simulink model "amplifierboard"  (R2020b)
settings: Solver=FixedStepDiscrete  StartTime=0.0  StopTime=2  FixedStep=0.01  RelTol=1e-3
InitFcn:
  | mbd_s32k_consistency_checks(bdroot(gcs));
undefined symbols (not defined in the file): AutoLowerVal, AutoRaiseVal, HoldVal, LED_En, LED_Off, LED_On, Logic_High, Logic_Low, LQFP, ManualLowerVal, ManualRaiseVal, PWRWNDW_CHDLCK, sC_bool_PWMEN, sC_cnt_FWSetting, sC_cnt_Mtr_DrvNo_HB, sC_cnt_PWMHB1to4, sC_cnt_PWMHB5to8, sC_cnt_TargetSlowRange, sC_pct_ManualMax, sC_pct_RampDwn, sC_pct_RampUp, sC_pct_StartPWM, sC_pct_Targetmax, SwitchPackRangeOffset, Threshold_Value, Tolerant_Time
libraries: mbd_s32k1xx_ec_toolbox x205, simulink x59, canmsglib x19, Filter x15, wndwcmd x3
(part 3 of 6)

== system amplifierboard/Initialization- Memory Defines/Generate_Data2 ==
  Constant2 : Constant  Value=3  OutDataTypeStr=uint8
  Constant{3,5..6,8} (4 alike) : Constant  Value=2  OutDataTypeStr=uint8
  Constant4 : Constant  OutDataTypeStr=uint8
  Constant7 : Constant  OutDataTypeStr=uint8
  Data Store Read1 : DataStoreRead  DataStoreName=data2
  Mux : Mux  Inputs=8
  Width : Width  DataType=uint8
  Data : Outport
  Length : Outport  Port=2
  wires:
  Mux/1 -> Width/1, Data/1
  Constant2/1 -> Mux/1
  Constant3/1 -> Mux/2
  Constant5/1 -> Mux/4
  Data Store Read1/1 -> Mux/5
  Constant4/1 -> Mux/3
  Constant6/1 -> Mux/6
  Constant7/1 -> Mux/7
  Constant8/1 -> Mux/8
  Width/1 -> Length/1

== system amplifierboard/Initialization- Memory Defines/Generate_Data3 ==
  Constant2 : Constant  Value=3  OutDataTypeStr=uint8
  Constant{3,5..6,8} (4 alike) : Constant  Value=2  OutDataTypeStr=uint8
  Constant4 : Constant  OutDataTypeStr=uint8
  Constant7 : Constant  OutDataTypeStr=uint8
  Data Store Read1 : DataStoreRead  DataStoreName=data3
  Mux : Mux  Inputs=8
  Width : Width  DataType=uint8
  Data : Outport
  Length : Outport  Port=2
  wires:
  Mux/1 -> Width/1, Data/1
  Constant2/1 -> Mux/1
  Constant3/1 -> Mux/2
  Constant5/1 -> Mux/4
  Data Store Read1/1 -> Mux/5
  Constant4/1 -> Mux/3
  Constant6/1 -> Mux/6
  Constant7/1 -> Mux/7
  Constant8/1 -> Mux/8
  Width/1 -> Length/1

== system amplifierboard/Initialization- Memory Defines/Generate_Data4 ==
  Constant2 : Constant  Value=3  OutDataTypeStr=uint8
  Constant{3,5..6,8} (4 alike) : Constant  Value=2  OutDataTypeStr=uint8
  Constant4 : Constant  OutDataTypeStr=uint8
  Constant7 : Constant  OutDataTypeStr=uint8
  Data Store Read1 : DataStoreRead  DataStoreName=data5
  Mux : Mux  Inputs=8
  Width : Width  DataType=uint8
  Data : Outport
  Length : Outport  Port=2
  wires:
  Width/1 -> Length/1
  Constant8/1 -> Mux/8
  Constant7/1 -> Mux/7
  Constant6/1 -> Mux/6
  Constant4/1 -> Mux/3
  Data Store Read1/1 -> Mux/5
  Constant5/1 -> Mux/4
  Constant3/1 -> Mux/2
  Constant2/1 -> Mux/1
  Mux/1 -> Data/1, Width/1

== system amplifierboard/Initialization- Memory Defines/Generate_Data5 ==
  Constant2 : Constant  Value=3  OutDataTypeStr=uint8
  Constant{3,5..6,8} (4 alike) : Constant  Value=2  OutDataTypeStr=uint8
  Constant4 : Constant  OutDataTypeStr=uint8
  Constant7 : Constant  OutDataTypeStr=uint8
  Data Store Read1 : DataStoreRead  DataStoreName=data4
  Mux : Mux  Inputs=8
  Width : Width  DataType=uint8
  Data : Outport
  Length : Outport  Port=2
  wires:
  Mux/1 -> Width/1, Data/1
  Constant2/1 -> Mux/1
  Constant3/1 -> Mux/2
  Constant5/1 -> Mux/4
  Data Store Read1/1 -> Mux/5
  Constant4/1 -> Mux/3
  Constant6/1 -> Mux/6
  Constant7/1 -> Mux/7
  Constant8/1 -> Mux/8
  Width/1 -> Length/1

== system amplifierboard/Initialization- Memory Defines/Generate_Data6 ==
  Constant2 : Constant  Value=3  OutDataTypeStr=uint8
  Constant{3,5..6,8} (4 alike) : Constant  Value=2  OutDataTypeStr=uint8
  Constant4 : Constant  OutDataTypeStr=uint8
  Constant7 : Constant  OutDataTypeStr=uint8
  Data Store Read1 : DataStoreRead  DataStoreName=data6
  Mux : Mux  Inputs=8
  Width : Width  DataType=uint8
  Data : Outport
  Length : Outport  Port=2
  wires:
  Mux/1 -> Width/1, Data/1
  Constant2/1 -> Mux/1
  Constant3/1 -> Mux/2
  Constant5/1 -> Mux/4
  Data Store Read1/1 -> Mux/5
  Constant4/1 -> Mux/3
  Constant6/1 -> Mux/6
  Constant7/1 -> Mux/7
  Constant8/1 -> Mux/8
  Width/1 -> Length/1

== system amplifierboard/Initialization- Memory Defines/Generate_Data7 ==
  Constant2 : Constant  OutDataTypeStr=uint8
  Constant3 : Constant  OutDataTypeStr=uint8
  Constant{4..8} (5 alike) : Constant  Value=85  OutDataTypeStr=uint8
  Data Store Read1 : DataStoreRead  DataStoreName=data6
  Mux : Mux  Inputs=8
  Width : Width  DataType=uint8
  Data : Outport
  Length : Outport  Port=2
  wires:
  Mux/1 -> Width/1, Data/1
  Constant2/1 -> Mux/1
  Constant3/1 -> Mux/2
  Constant5/1 -> Mux/4
  Data Store Read1/1 -> Mux/5
  Constant4/1 -> Mux/3
  Constant6/1 -> Mux/6
  Constant7/1 -> Mux/7
  Constant8/1 -> Mux/8
  Width/1 -> Length/1

== system amplifierboard/Initialization- Memory Defines/Subsystem ==
  FLASH_Config : mbd_s32k1xx_ec_toolbox/Core and System Blocks/FLASH Blocks/FLASH_Config  depart=0x2  eeesize=4096  csec_en=off  csec_num_user_keys=5 keys
  FLASH_EEERead : mbd_s32k1xx_ec_toolbox/Core and System Blocks/FLASH Blocks/FLASH_EEERead  base=0x14000000  offset=0x0F00  ptr=uint16_t
  FLASH_EEERead6 : mbd_s32k1xx_ec_toolbox/Core and System Blocks/FLASH Blocks/FLASH_EEERead  base=0x14000000  offset=0x0F0C  ptr=uint16_t
  If : If  NumInputs=2  IfExpression=(u1 <= 1200) & (u2 <= 750)
  If Action Subsystem : Subsystem  TreatAsAtomicUnit=on
  If Action Subsystem1 : Subsystem  TreatAsAtomicUnit=on  mask{sC_WindSw_NormOpen=1072, sC_WindSw_Dwn=680, sC_WindSw_ExpDwn=437, sC_WindSw_Up=257, sC_WindSw_ExpUp=114}
  wires:
  If/2 -> If Action Subsystem1/Action
  If/1 -> If Action Subsystem/Action
  FLASH_EEERead/1 -> If/1
  FLASH_EEERead6/1 -> If/2

== system amplifierboard/Motor_Control/Motor_Control ==
  note: MotorDir Index
      | Motor
      | Driver
      | HB
      | DRV_SO
      |
      | PWM
      | PWM_Pin
      | PWM FTM CH
      |
      | 1
      | Motor1
      | DRV1
      | 1,2
      | DRV1_SO_1
      |
      | DRV1_PWM1
      | PTA17
      | FTM0_CH6
      |
      | 2
      | Motor2
      | DRV1
      | 3,4
      | DRV1_SO_2
      |
      | DRV1_PWM2
      | PTA11
      | FTM1_CH5
      |
      | 3
      | Motor3
      | DRV1
      | 5,6
      | DRV2_SO_2
      |
      | DRV1_PWM3
      | PTA12
      | FTM1_CH6
      |
      | 4
      | Motor4
      | DRV1
      | 7,8
      | DRV2_SO_1
      |
      | DRV1_PWM4
      | PTA13
      | FTM1_CH7
      |
      | 5
      | Motor5
      | DRV2
      | 1,2
      | DRV3_SO_2
      |
      | DRV2_PWM1
      | PTB17
      | FTM0_CH5
      |
      | 6
      | Motor6
      | DRV2
      | 3,4
      | DRV3_SO_1
      |
      | DRV2_PWM2
      | PTB9
      | FTM3_CH1
      |
      | Shared Channels -None
  cMM_aV_int_MotorDir : Inport  OutDataTypeStr=int8  PortDimensions=6
  BRAKE1 : mbd_s32k1xx_ec_toolbox/GPIO Blocks/Digital_Output  gpio_pin=PTA8: [PTA8 | Port A I/O]  init_val=High  drive_strength=High
  BRAKE2 : mbd_s32k1xx_ec_toolbox/GPIO Blocks/Digital_Output  gpio_pin=PTA0: [PTA0 | Port A I/O]  init_val=High  drive_strength=High
  Chart : Stateflow chart  TreatAsAtomicUnit=on
  Constant : Constant  Value=sC_cnt_PWMHB1to4
  Constant1 : Constant  Value=sC_cnt_PWMHB5to8
  Constant2 : Constant  Value=sC_cnt_Mtr_DrvNo_HB
  Constant3 : Constant  Value=sC_bool_PWMEN
  Constant4 : Constant  Value=sC_cnt_FWSetting  OutDataTypeStr=uint8
  Constant{5..8} (4 alike) : Constant  OutDataTypeStr=Inherit: Inherit via back propagation
  Digital_Output : mbd_s32k1xx_ec_toolbox/GPIO Blocks/Digital_Output  gpio_pin=PTE0: [PTE0 | Port E I/O]  init_val=High  drive_strength=High
  Digital_Output1 : mbd_s32k1xx_ec_toolbox/GPIO Blocks/Digital_Output  gpio_pin=PTB8: [PTB8 | Port B I/O]  init_val=High  drive_strength=High
  "LPSPI_Config " : mbd_s32k1xx_ec_toolbox/Communication Blocks/SPI Blocks/LPSPI_Config   Priority=0  InstanceNumber=2  Role=Master  BaudRate=10000  ShowAdvanced=on  sin=PTC0: [LPSPI2_SIN | LPSPI Serial Data Input]  sout=PTC1: [LPSPI2_SOUT | LPSPI Serial Data Output]  sck=PTC15: [LPSPI2_SCK | LPSPI Serial Clock I/O]  pcs0=PTE11: [LPSPI2_PCS0 | Peripheral Chip Select 0]  pcs1=None  pcs2=None  pcs3=None  CPHA=1  CPOL=0  BitOrder=MSB first  TransferSize=8  WhichPCS=0  PCSPol=ActiveLow  ContinuousTransfer=on
  LPSPI_Config 1 : mbd_s32k1xx_ec_toolbox/Communication Blocks/SPI Blocks/LPSPI_Config   Priority=0  InstanceNumber=1  Role=Master  BaudRate=10000  ShowAdvanced=on  sin=PTD1: [LPSPI1_SIN | LPSPI Serial Data Input]  sout=PTB16: [LPSPI1_SOUT | LPSPI Serial Data Output]  sck=PTD0: [LPSPI1_SCK | LPSPI Serial Clock I/O]  pcs0=None  pcs1=PTA6: [LPSPI1_PCS1 | Peripheral Chip Select 1]  pcs2=None  pcs3=None  CPHA=1  CPOL=0  BitOrder=MSB first  TransferSize=8  WhichPCS=0  PCSPol=ActiveLow  ContinuousTransfer=on
  nSLEEP1 : mbd_s32k1xx_ec_toolbox/GPIO Blocks/Digital_Output  gpio_pin=PTA9: [PTA9 | Port A I/O]  init_val=High  drive_strength=High
  nSLEEP2 : mbd_s32k1xx_ec_toolbox/GPIO Blocks/Digital_Output  gpio_pin=PTA1: [PTA1 | Port A I/O]  init_val=High  drive_strength=High
  8718_FailSafe : Outport
  MotorDriverState : Outport  Port=2
  wires:
  Chart/1(DRV1_OFF) -> Digital_Output/1
  Chart/2(DRV2_OFF) -> Digital_Output1/1
  Constant/1 -> Chart/2(sC_cnt_PWMHB1to4)
  Constant1/1 -> Chart/3(sC_cnt_PWMHB5to8)
  Constant2/1 -> Chart/4(sC_cnt_Mtr_DrvNo_HB)
  Constant3/1 -> Chart/5(sC_bool_PWMEN)
  Constant4/1 -> Chart/6(sC_cnt_FWSetting)
  cMM_aV_int_MotorDir/1 -> Chart/1(aV_int_MotorDir)
  Constant7/1 -> nSLEEP1/1
  Constant6/1 -> BRAKE2/1
  Constant8/1 -> nSLEEP2/1
  Constant5/1 -> BRAKE1/1
  Chart/3(FailSafe) -> 8718_FailSafe/1
  Chart/4(MotorDriverState) -> MotorDriverState/1

== system amplifierboard/Motor_Control/Subsystem ==
  note: MotorDir Index
      | Motor
      | Driver
      | HB
      | DRV_SO
      |
      | PWM
      | PWM_Pin
      | PWM FTM CH
      |
      | 1
      | Motor1
      | DRV1
      | 1,2
      | DRV1_SO_1
      |
      | DRV1_PWM1
      | PTA17
      | FTM0_CH6
      |
      | 2
      | Motor2
      | DRV1
      | 3,4
      | DRV1_SO_2
      |
      | DRV1_PWM2
      | PTA11
      | FTM1_CH5
      |
      | 3
      | Motor3
      | DRV1
      | 5,6
      | DRV2_SO_2
      |
      | DRV1_PWM3
      | PTA12
      | FTM1_CH6
      |
      | 4
      | Motor4
      | DRV1
      | 7,8
      | DRV2_SO_1
      |
      | DRV1_PWM4
      | PTA13
      | FTM1_CH7
      |
      | 5
      | Motor5
      | DRV2
      | 1,2
      | DRV3_SO_2
      |
      | DRV2_PWM1
      | PTB17
      | FTM0_CH5
      |
      | 6
      | Motor6
      | DRV2
      | 3,4
      | DRV3_SO_1
      |
      | DRV2_PWM2
      | PTB9
      | FTM3_CH1
      |
      | Shared Channels -None
  cMM_aV_int_MotorDir1 : Inport  OutDataTypeStr=int8  PortDimensions=6
  cMM_aV_int_PositionError : Inport  Port=2  OutDataTypeStr=uint8  PortDimensions=6
  Abs : Abs
  Chart : Stateflow chart  TreatAsAtomicUnit=on
  Constant : Constant  Value=sC_pct_RampUp  OutDataTypeStr=single
  Constant1 : Constant  Value=sC_pct_RampDwn  OutDataTypeStr=single
  Constant2 : Constant  Value=sC_pct_StartPWM  OutDataTypeStr=single
  Constant3 : Constant  Value=sC_pct_ManualMax  OutDataTypeStr=single
  Constant4 : Constant  Value=sC_pct_Targetmax  OutDataTypeStr=single
  Constant5 : Constant  Value=sC_cnt_TargetSlowRange  OutDataTypeStr=uint16
  aV_pct_PWMOut1 : Outport  OutDataTypeStr=single  PortDimensions=6
  wires:
  Abs/1 -> Chart/1(aV_int_MotorDir)
  Constant1/1 -> Chart/4(RampDwn)
  Constant3/1 -> Chart/6(ManualMaxPWM)
  Constant4/1 -> Chart/7(TargetMaxPWM)
  Constant5/1 -> Chart/8(TargetSlowRange)
  Constant2/1 -> Chart/5(StartPWM)
  cMM_aV_int_MotorDir1/1 -> Abs/1
  Constant/1 -> Chart/3(RampUp)
  Chart/1(PWM_Out) -> aV_pct_PWMOut1/1
  cMM_aV_int_PositionError/1 -> Chart/2(PositionError)

== system amplifierboard/TC1047A_Module/temperature_conversion ==
  In1 : Inport
  Constant1 : Constant  Value=273
  Data Type Conversion : DataTypeConversion
  Degree_to_Kelvin : Sum
  Divide : Product  Inputs=*/  RndMeth=Zero  SaturateOnIntegerOverflow=on
  Divide1 : Product  Inputs=*/  RndMeth=Zero  SaturateOnIntegerOverflow=on
  Divide2 : Product  Inputs=**  RndMeth=Zero  SaturateOnIntegerOverflow=on
  Subtract : Sum  Inputs=+-
  adc_resolution_val : Constant  Value=4095
  adc_vref_val : Constant  Value=5
  mv_to_temp_factor_val : Constant  Value=0.01
  temp_offset_factor_val : Constant  Value=0.5
  AmpBoard_PRV_CAN_Msg_TX_TMP : Outport
  wires:
  Subtract/1 -> Divide/1
  Divide2/1 -> Subtract/1
  In1/1 -> Data Type Conversion/1
  adc_resolution_val/1 -> Divide1/2
  Data Type Conversion/1 -> Divide1/1
  mv_to_temp_factor_val/1 -> Divide/2
  Divide1/1 -> Divide2/1
  adc_vref_val/1 -> Divide2/2
  temp_offset_factor_val/1 -> Subtract/2
  Divide/1 -> Degree_to_Kelvin/1
  Constant1/1 -> Degree_to_Kelvin/2
  Degree_to_Kelvin/1 -> AmpBoard_PRV_CAN_Msg_TX_TMP/1

== system amplifierboard/CAN_Pack_And_Send/PsngrWndwCntDetect/SwtchPosDetect ==
  SwitchCount : Inport
  FR_Dwn_CntDetect : Subsystem
  FR_ExpDwn_CntDetect : Subsystem
  FR_ExpUp_CntDetect : Subsystem
  FR_NrmOpen_CntDetect : Subsystem
  FR_Up_CntDetect : Subsystem
  SwitchPosDetect : Subsystem
  AvgCount : Outport
  wires:
  FR_NrmOpen_CntDetect/1(HoldCnt) -> SwitchPosDetect/5(HoldCnt)  "HoldCnt"
  SwitchPosDetect/1(AvgCount) -> AvgCount/1  "AvgCount"
  FR_ExpDwn_CntDetect/1(Out) -> SwitchPosDetect/4(AutoLowerCnt)  "AutoLowerCnt"
  FR_Dwn_CntDetect/1(Out1) -> SwitchPosDetect/2(ManLowerCnt)  "ManLowerCnt"
  FR_Up_CntDetect/1(Out3) -> SwitchPosDetect/1(ManRaiseCnt)  "ManRaiseCnt"
  SwitchCount/1 -> FR_Up_CntDetect/1(In3), FR_Dwn_CntDetect/1(In1), FR_ExpUp_CntDetect/1(In2), FR_ExpDwn_CntDetect/1(In), FR_NrmOpen_CntDetect/1(In4), SwitchPosDetect/6(SwitchCount)  "SwitchCount"
  FR_ExpUp_CntDetect/1(AutoRaiseCnt) -> SwitchPosDetect/3(AutoRaiseCnt)

== system amplifierboard/CAN_Pack_And_Send/RLWndwCntDetect/SwtchPosDetect ==
  SwitchCount : Inport
  RL_Dwn_CntDetect : Subsystem
  RL_ExpDwn_CntDetect : Subsystem
  RL_ExpUp_CntDetect : Subsystem
  RL_NrmOpen_CntDetect : Subsystem
  RL_Up_CntDetect : Subsystem
  SwitchPosDetect2 : Subsystem
  AvgCount : Outport
  wires:
  SwitchPosDetect2/1(AvgCount) -> AvgCount/1  "AvgCount"
  SwitchCount/1 -> RL_Up_CntDetect/1(In13), RL_Dwn_CntDetect/1(In11), RL_ExpUp_CntDetect/1(In12), RL_ExpDwn_CntDetect/1(In10), RL_NrmOpen_CntDetect/1(In14), SwitchPosDetect2/6(SwitchCount)
  RL_Up_CntDetect/1(Out13) -> SwitchPosDetect2/1(ManRaiseCnt)  "ManRaiseCnt"
  RL_ExpUp_CntDetect/1(Out12) -> SwitchPosDetect2/3(AutoRaiseCnt)
  RL_Dwn_CntDetect/1(ManLowerCnt) -> SwitchPosDetect2/2(ManLowerCnt)
  RL_ExpDwn_CntDetect/1(AutoLowerCnt) -> SwitchPosDetect2/4(AutoLowerCnt)
  RL_NrmOpen_CntDetect/1(HoldCnt) -> SwitchPosDetect2/5(HoldCnt)

== system amplifierboard/CAN_Pack_And_Send/RRWndwCntDetect/SwtchPosDetect ==
  SwitchCount : Inport
  RR_Dwn_CntDetect : Subsystem
  RR_ExpDwn_CntDetect : Subsystem
  RR_ExpUp_CntDetect : Subsystem
  RR_NrmOpen_CntDetect : Subsystem
  RR_Up_CntDetect : Subsystem
  SwitchPosDetect1 : Subsystem
  AvgCount : Outport
  wires:
  RR_Up_CntDetect/1(Out8) -> SwitchPosDetect1/1(ManRaiseCnt)  "ManRaiseCnt"
  RR_Dwn_CntDetect/1(Out6) -> SwitchPosDetect1/2(ManLowerCnt)  "ManLowerCnt"
  RR_ExpDwn_CntDetect/1(Out5) -> SwitchPosDetect1/4(AutoLowerCnt)  "AutoLowerCnt"
  RR_ExpUp_CntDetect/1(AutoRaiseCnt) -> SwitchPosDetect1/3(AutoRaiseCnt)
  SwitchCount/1 -> RR_Up_CntDetect/1(In8), RR_Dwn_CntDetect/1(In6), RR_ExpUp_CntDetect/1(In7), RR_ExpDwn_CntDetect/1(SwitchCount1), RR_NrmOpen_CntDetect/1(In9), SwitchPosDetect1/6(SwitchCount)
  SwitchPosDetect1/1(AvgCount) -> AvgCount/1  "AvgCount"
  RR_NrmOpen_CntDetect/1(HoldCnt) -> SwitchPosDetect1/5(HoldCnt)

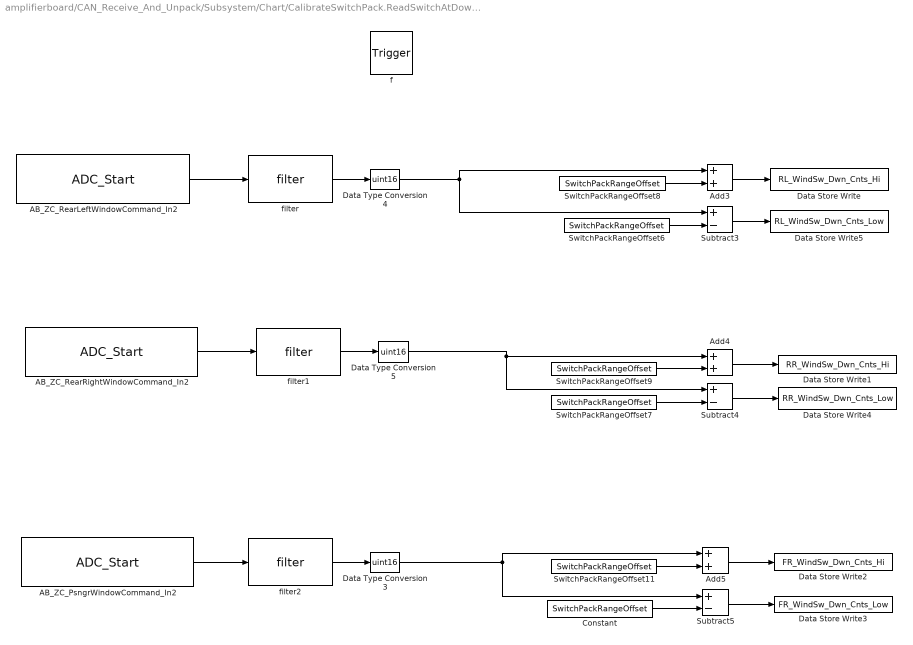
== system amplifierboard/CAN_Receive_And_Unpack/Subsystem/Chart/CalibrateSwitchPack.ReadSwitchAtDownPostion ==
  f : TriggerPort  TriggerType=function-call  VariantControl=(inherit)
      settings: CopyFcn=Stateflow.SLINSF.SimulinkMan.removeBlockPreDeleteFcn  PreDeleteFcn=Stateflow.SLINSF.SimulinkMan.unsafePredeleteFcn
  AB_ZC_PsngrWindowCommand_In2 : mbd_s32k1xx_ec_toolbox/Motor Control Blocks/ADC Blocks/ADC_Start  instance=0  adc_r=A  adc_chan=PTB2: [ADC0_SE6 | ADC Single Ended Input]  aien=off  mcuTargetUpdate=on
  AB_ZC_RearLeftWindowCommand_In2 : mbd_s32k1xx_ec_toolbox/Motor Control Blocks/ADC Blocks/ADC_Start  instance=0  adc_r=A  adc_chan=PTB0: [ADC0_SE4 | ADC Single Ended Input]  aien=off  mcuTargetUpdate=on
  AB_ZC_RearRightWindowCommand_In2 : mbd_s32k1xx_ec_toolbox/Motor Control Blocks/ADC Blocks/ADC_Start  instance=0  adc_r=A  adc_chan=PTB1: [ADC0_SE5 | ADC Single Ended Input]  aien=off  mcuTargetUpdate=on
  Add3 : Sum  OutDataTypeStr=uint16
  Add4 : Sum
  Add5 : Sum
  Constant : Constant  Value=SwitchPackRangeOffset  OutDataTypeStr=uint16
  Data Store Write : DataStoreWrite  DataStoreName=RL_WindSw_Dwn_Cnts_Hi
  Data Store Write1 : DataStoreWrite  DataStoreName=RR_WindSw_Dwn_Cnts_Hi
  Data Store Write2 : DataStoreWrite  DataStoreName=FR_WindSw_Dwn_Cnts_Hi
  Data Store Write3 : DataStoreWrite  DataStoreName=FR_WindSw_Dwn_Cnts_Low
  Data Store Write4 : DataStoreWrite  DataStoreName=RR_WindSw_Dwn_Cnts_Low
  Data Store Write5 : DataStoreWrite  DataStoreName=RL_WindSw_Dwn_Cnts_Low
  Data Type Conversion3 : DataTypeConversion  OutDataTypeStr=uint16
  Data Type Conversion4 : DataTypeConversion  OutDataTypeStr=uint16
  Data Type Conversion5 : DataTypeConversion  OutDataTypeStr=uint16
  Subtract3 : Sum  Inputs=+-
  Subtract4 : Sum  Inputs=+-
  Subtract5 : Sum  Inputs=+-
  SwitchPackRangeOffset{6..9,11} (5 alike) : Constant  Value=SwitchPackRangeOffset  OutDataTypeStr=uint16
  filter : Filter/filter  pwrwndwp_coefcnt=pwrwndwp_coefcnt
  filter1 : Filter/filter  pwrwndwp_coefcnt=pwrwndwp_coefcnt
  filter2 : Filter/filter  pwrwndwp_coefcnt=pwrwndwp_coefcnt
  wires:
  AB_ZC_PsngrWindowCommand_In2/1 -> filter2/1
  AB_ZC_RearRightWindowCommand_In2/1 -> filter1/1
  AB_ZC_RearLeftWindowCommand_In2/1 -> filter/1
  Constant/1 -> Subtract5/2
  SwitchPackRangeOffset11/1 -> Add5/2
  SwitchPackRangeOffset8/1 -> Add3/2
  SwitchPackRangeOffset6/1 -> Subtract3/2
  SwitchPackRangeOffset7/1 -> Subtract4/2
  Add4/1 -> Data Store Write1/1
  SwitchPackRangeOffset9/1 -> Add4/2
  Add5/1 -> Data Store Write2/1
  Subtract3/1 -> Data Store Write5/1
  Add3/1 -> Data Store Write/1
  Subtract4/1 -> Data Store Write4/1
  Subtract5/1 -> Data Store Write3/1
  Data Type Conversion3/1 -> Subtract5/1, Add5/1
  Data Type Conversion4/1 -> Add3/1, Subtract3/1
  Data Type Conversion5/1 -> Subtract4/1, Add4/1
  filter/1 -> Data Type Conversion4/1
  filter1/1 -> Data Type Conversion5/1
  filter2/1 -> Data Type Conversion3/1

== system amplifierboard/CAN_Receive_And_Unpack/Subsystem/Chart/CalibrateSwitchPack.ReadSwitchAtExpDownPosition ==
  f : TriggerPort  TriggerType=function-call  VariantControl=(inherit)
      settings: CopyFcn=Stateflow.SLINSF.SimulinkMan.removeBlockPreDeleteFcn  PreDeleteFcn=Stateflow.SLINSF.SimulinkMan.unsafePredeleteFcn
  AB_ZC_PsngrWindowCommand_In1 : mbd_s32k1xx_ec_toolbox/Motor Control Blocks/ADC Blocks/ADC_Start  instance=0  adc_r=A  adc_chan=PTB2: [ADC0_SE6 | ADC Single Ended Input]  aien=off  mcuTargetUpdate=on
  AB_ZC_RearLeftWindowCommand_In1 : mbd_s32k1xx_ec_toolbox/Motor Control Blocks/ADC Blocks/ADC_Start  instance=0  adc_r=A  adc_chan=PTB0: [ADC0_SE4 | ADC Single Ended Input]  aien=off  mcuTargetUpdate=on
  AB_ZC_RearRightWindowCommand_In1 : mbd_s32k1xx_ec_toolbox/Motor Control Blocks/ADC Blocks/ADC_Start  instance=0  adc_r=A  adc_chan=PTB1: [ADC0_SE5 | ADC Single Ended Input]  aien=off  mcuTargetUpdate=on
  Add1 : Sum
  Add2 : Sum  OutDataTypeStr=uint16
  Add6 : Sum  OutDataTypeStr=uint16
  Data Store Write10 : DataStoreWrite  DataStoreName=RR_WindSw_ExpDwn_Cnts_Hi
  Data Store Write11 : DataStoreWrite  DataStoreName=FR_WindSw_ExpDwn_Cnts_Hi
  Data Store Write6 : DataStoreWrite  DataStoreName=FR_WindSw_ExpDwn_Cnts_Low
  Data Store Write7 : DataStoreWrite  DataStoreName=RR_WindSw_ExpDwn_Cnts_Low
  Data Store Write8 : DataStoreWrite  DataStoreName=RL_WindSw_ExpDwn_Cnts_Hi
  Data Store Write9 : DataStoreWrite  DataStoreName=RL_WindSw_ExpDwn_Cnts_Low
  Data Type Conversion2 : DataTypeConversion  OutDataTypeStr=uint16
  Data Type Conversion3 : DataTypeConversion  OutDataTypeStr=uint16
  Data Type Conversion5 : DataTypeConversion  OutDataTypeStr=uint16
  Subtract1 : Sum  Inputs=+-
  Subtract2 : Sum  Inputs=+-  OutDataTypeStr=uint16
  Subtract6 : Sum  Inputs=+-  OutDataTypeStr=uint16
  SwitchPackRangeOffset1 : Constant  Value=SwitchPackRangeOffset  OutDataTypeStr=uint16
  SwitchPackRangeOffset{3..5,12} (4 alike) : Constant  Value=SwitchPackRangeOffset  OutDataTypeStr=Inherit: Inherit via back propagation
  SwitchPackRangeOffset2 : Constant  Value=SwitchPackRangeOffset  OutDataTypeStr=uint16
  filter : Filter/filter  pwrwndwp_coefcnt=pwrwndwp_coefcnt
  filter1 : Filter/filter  pwrwndwp_coefcnt=pwrwndwp_coefcnt
  filter2 : Filter/filter  pwrwndwp_coefcnt=pwrwndwp_coefcnt
  wires:
  AB_ZC_RearLeftWindowCommand_In1/1 -> filter/1
  AB_ZC_RearRightWindowCommand_In1/1 -> filter1/1
  Subtract6/1 -> Data Store Write6/1
  SwitchPackRangeOffset4/1 -> Subtract2/2
  Subtract1/1 -> Data Store Write9/1
  SwitchPackRangeOffset3/1 -> Subtract1/2
  SwitchPackRangeOffset1/1 -> Subtract6/2
  SwitchPackRangeOffset2/1 -> Add6/2
  Add2/1 -> Data Store Write10/1
  Add6/1 -> Data Store Write11/1
  SwitchPackRangeOffset5/1 -> Add1/2
  Subtract2/1 -> Data Store Write7/1
  SwitchPackRangeOffset12/1 -> Add2/2
  Add1/1 -> Data Store Write8/1
  Data Type Conversion3/1 -> Subtract1/1, Add1/1
  Data Type Conversion2/1 -> Subtract2/1, Add2/1
  Data Type Conversion5/1 -> Add6/1, Subtract6/1
  filter/1 -> Data Type Conversion3/1
  filter1/1 -> Data Type Conversion2/1
  filter2/1 -> Data Type Conversion5/1
  AB_ZC_PsngrWindowCommand_In1/1 -> filter2/1

== system amplifierboard/CAN_Receive_And_Unpack/Subsystem/Chart/CalibrateSwitchPack.ReadSwitchAtExpUpPosition ==
  f : TriggerPort  TriggerType=function-call  VariantControl=(inherit)
      settings: CopyFcn=Stateflow.SLINSF.SimulinkMan.removeBlockPreDeleteFcn  PreDeleteFcn=Stateflow.SLINSF.SimulinkMan.unsafePredeleteFcn
  AB_ZC_PsngrWindowCommand_In4 : mbd_s32k1xx_ec_toolbox/Motor Control Blocks/ADC Blocks/ADC_Start  instance=0  adc_r=A  adc_chan=PTB2: [ADC0_SE6 | ADC Single Ended Input]  aien=off  mcuTargetUpdate=on
  AB_ZC_RearLeftWindowCommand_In4 : mbd_s32k1xx_ec_toolbox/Motor Control Blocks/ADC Blocks/ADC_Start  instance=0  adc_r=A  adc_chan=PTB0: [ADC0_SE4 | ADC Single Ended Input]  aien=off  mcuTargetUpdate=on
  AB_ZC_RearRightWindowCommand_In4 : mbd_s32k1xx_ec_toolbox/Motor Control Blocks/ADC Blocks/ADC_Start  instance=0  adc_r=A  adc_chan=PTB1: [ADC0_SE5 | ADC Single Ended Input]  aien=off  mcuTargetUpdate=on
  Add1 : Sum
  Add2 : Sum
  Add6 : Sum
  Data Store Write12 : DataStoreWrite  DataStoreName=RL_WindSw_ExpUp_Cnts_Low
  Data Store Write2 : DataStoreWrite  DataStoreName=RR_WindSw_ExpUp_Cnts_Hi
  Data Store Write3 : DataStoreWrite  DataStoreName=FR_WindSw_ExpUp_Cnts_Hi
  Data Store Write6 : DataStoreWrite  DataStoreName=FR_WindSw_ExpUp_Cnts_Low
  Data Store Write7 : DataStoreWrite  DataStoreName=RR_WindSw_ExpUp_Cnts_Low
  Data Store Write8 : DataStoreWrite  DataStoreName=RL_WindSw_ExpUp_Cnts_Hi
  Data Type Conversion3 : DataTypeConversion  OutDataTypeStr=uint16
  Data Type Conversion4 : DataTypeConversion  OutDataTypeStr=uint16
  Data Type Conversion6 : DataTypeConversion  OutDataTypeStr=uint16
  Subtract1 : Sum  Inputs=+-
  Subtract2 : Sum  Inputs=+-
  Subtract6 : Sum  Inputs=+-
  SwitchPackRangeOffset{1..5,12} (6 alike) : Constant  Value=SwitchPackRangeOffset  OutDataTypeStr=uint16
  filter : Filter/filter  pwrwndwp_coefcnt=pwrwndwp_coefcnt
  filter1 : Filter/filter  pwrwndwp_coefcnt=pwrwndwp_coefcnt
  filter2 : Filter/filter  pwrwndwp_coefcnt=pwrwndwp_coefcnt
  wires:
  AB_ZC_PsngrWindowCommand_In4/1 -> filter2/1
  AB_ZC_RearRightWindowCommand_In4/1 -> filter1/1
  AB_ZC_RearLeftWindowCommand_In4/1 -> filter/1
  Data Type Conversion6/1 -> Add6/1, Subtract6/1
  Subtract2/1 -> Data Store Write7/1
  SwitchPackRangeOffset5/1 -> Add1/2
  SwitchPackRangeOffset3/1 -> Subtract1/2
  SwitchPackRangeOffset4/1 -> Subtract2/2
  Add1/1 -> Data Store Write8/1
  Data Type Conversion4/1 -> Add2/1, Subtract2/1
  Data Type Conversion3/1 -> Add1/1, Subtract1/1
  SwitchPackRangeOffset2/1 -> Add6/2
  Subtract6/1 -> Data Store Write6/1
  SwitchPackRangeOffset12/1 -> Add2/2
  SwitchPackRangeOffset1/1 -> Subtract6/2
  Add6/1 -> Data Store Write3/1
  Add2/1 -> Data Store Write2/1
  Subtract1/1 -> Data Store Write12/1
  filter/1 -> Data Type Conversion3/1
  filter1/1 -> Data Type Conversion4/1
  filter2/1 -> Data Type Conversion6/1

== system amplifierboard/CAN_Receive_And_Unpack/Subsystem/Chart/CalibrateSwitchPack.ReadSwitchAtNormOpen ==
  f : TriggerPort  TriggerType=function-call  VariantControl=(inherit)
      settings: CopyFcn=Stateflow.SLINSF.SimulinkMan.removeBlockPreDeleteFcn  PreDeleteFcn=Stateflow.SLINSF.SimulinkMan.unsafePredeleteFcn
  AB_ZC_PsngrWindowCommand_In4 : mbd_s32k1xx_ec_toolbox/Motor Control Blocks/ADC Blocks/ADC_Start  instance=0  adc_r=A  adc_chan=PTB2: [ADC0_SE6 | ADC Single Ended Input]  aien=off  mcuTargetUpdate=on
  AB_ZC_RearLeftWindowCommand_In4 : mbd_s32k1xx_ec_toolbox/Motor Control Blocks/ADC Blocks/ADC_Start  instance=0  adc_r=A  adc_chan=PTB0: [ADC0_SE4 | ADC Single Ended Input]  aien=off  mcuTargetUpdate=on
  AB_ZC_RearRightWindowCommand_In4 : mbd_s32k1xx_ec_toolbox/Motor Control Blocks/ADC Blocks/ADC_Start  instance=0  adc_r=A  adc_chan=PTB1: [ADC0_SE5 | ADC Single Ended Input]  aien=off  mcuTargetUpdate=on
  Add : Sum
  Add1 : Sum
  Add2 : Sum
  Data Store Write12 : DataStoreWrite  DataStoreName=RL_WindSw_NrmOpen_Cnts_Low
  Data Store Write13 : DataStoreWrite  DataStoreName=RR_WindSw_NrmOpen_Cnts_Low
  Data Store Write14 : DataStoreWrite  DataStoreName=FR_WindSw_NrmOpen_Cnts_Low
  Data Store Write6 : DataStoreWrite  DataStoreName=FR_WindSw_NrmOpen_Cnts_Hi
  Data Store Write7 : DataStoreWrite  DataStoreName=RR_WindSw_NrmOpen_Cnts_Hi
  Data Store Write8 : DataStoreWrite  DataStoreName=RL_WindSw_NrmOpen_Cnts_Hi
  Data Type Conversion2 : DataTypeConversion  OutDataTypeStr=uint16
  Data Type Conversion3 : DataTypeConversion  OutDataTypeStr=uint16
  Data Type Conversion4 : DataTypeConversion  OutDataTypeStr=uint16
  Subtract : Sum  Inputs=+-
  Subtract1 : Sum  Inputs=+-
  Subtract2 : Sum  Inputs=+-
  SwitchPackRangeOffset{,1..5} (6 alike) : Constant  Value=SwitchPackRangeOffset  OutDataTypeStr=uint16
  filter : Filter/filter  pwrwndwp_coefcnt=pwrwndwp_coefcnt
  filter1 : Filter/filter  pwrwndwp_coefcnt=pwrwndwp_coefcnt
  filter2 : Filter/filter  pwrwndwp_coefcnt=pwrwndwp_coefcnt
  wires:
  AB_ZC_PsngrWindowCommand_In4/1 -> filter2/1
  AB_ZC_RearRightWindowCommand_In4/1 -> filter1/1
  AB_ZC_RearLeftWindowCommand_In4/1 -> filter/1
  SwitchPackRangeOffset2/1 -> Add/2
  Add/1 -> Data Store Write8/1
  Subtract/1 -> Data Store Write12/1
  SwitchPackRangeOffset/1 -> Subtract/2
  SwitchPackRangeOffset1/1 -> Subtract1/2
  Subtract1/1 -> Data Store Write13/1
  Add1/1 -> Data Store Write7/1
  SwitchPackRangeOffset3/1 -> Add1/2
  filter1/1 -> Data Type Conversion4/1
  SwitchPackRangeOffset4/1 -> Subtract2/2
  Subtract2/1 -> Data Store Write14/1
  SwitchPackRangeOffset5/1 -> Add2/2
  Add2/1 -> Data Store Write6/1
  filter/1 -> Data Type Conversion3/1
  Data Type Conversion2/1 -> Add2/1, Subtract2/1
  Data Type Conversion4/1 -> Add1/1, Subtract1/1
  Data Type Conversion3/1 -> Add/1, Subtract/1
  filter2/1 -> Data Type Conversion2/1

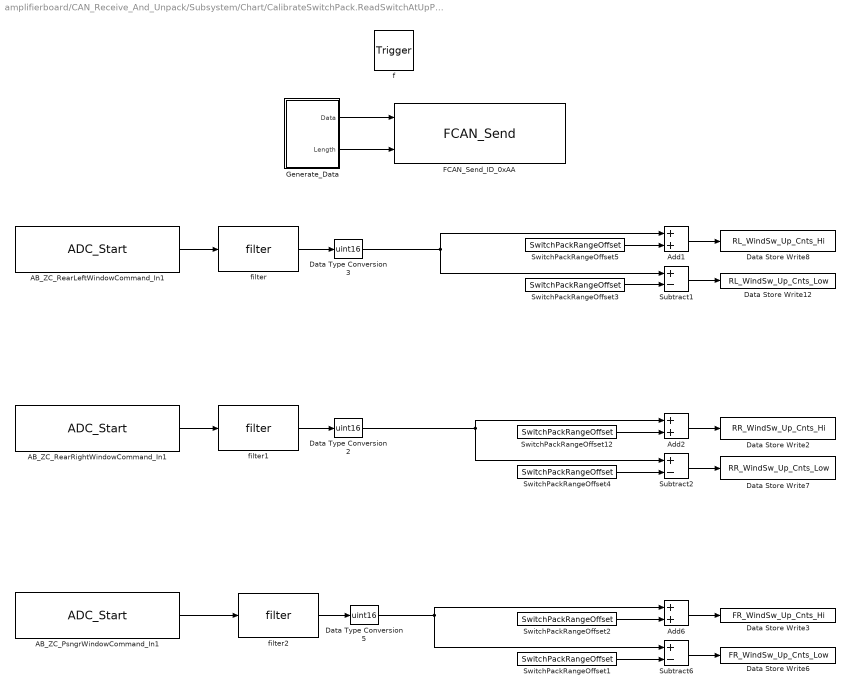
== system amplifierboard/CAN_Receive_And_Unpack/Subsystem/Chart/CalibrateSwitchPack.ReadSwitchAtUpPosition ==
  f : TriggerPort  TriggerType=function-call  VariantControl=(inherit)
      settings: CopyFcn=Stateflow.SLINSF.SimulinkMan.removeBlockPreDeleteFcn  PreDeleteFcn=Stateflow.SLINSF.SimulinkMan.unsafePredeleteFcn
  AB_ZC_PsngrWindowCommand_In1 : mbd_s32k1xx_ec_toolbox/Motor Control Blocks/ADC Blocks/ADC_Start  instance=0  adc_r=A  adc_chan=PTB2: [ADC0_SE6 | ADC Single Ended Input]  aien=off  mcuTargetUpdate=on
  AB_ZC_RearLeftWindowCommand_In1 : mbd_s32k1xx_ec_toolbox/Motor Control Blocks/ADC Blocks/ADC_Start  instance=0  adc_r=A  adc_chan=PTB0: [ADC0_SE4 | ADC Single Ended Input]  aien=off  mcuTargetUpdate=on
  AB_ZC_RearRightWindowCommand_In1 : mbd_s32k1xx_ec_toolbox/Motor Control Blocks/ADC Blocks/ADC_Start  instance=0  adc_r=A  adc_chan=PTB1: [ADC0_SE5 | ADC Single Ended Input]  aien=off  mcuTargetUpdate=on
  Add1 : Sum
  Add2 : Sum
  Add6 : Sum
  Data Store Write12 : DataStoreWrite  DataStoreName=RL_WindSw_Up_Cnts_Low
  Data Store Write2 : DataStoreWrite  DataStoreName=RR_WindSw_Up_Cnts_Hi
  Data Store Write3 : DataStoreWrite  DataStoreName=FR_WindSw_Up_Cnts_Hi
  Data Store Write6 : DataStoreWrite  DataStoreName=FR_WindSw_Up_Cnts_Low
  Data Store Write7 : DataStoreWrite  DataStoreName=RR_WindSw_Up_Cnts_Low
  Data Store Write8 : DataStoreWrite  DataStoreName=RL_WindSw_Up_Cnts_Hi
  Data Type Conversion2 : DataTypeConversion  OutDataTypeStr=uint16
  Data Type Conversion3 : DataTypeConversion  OutDataTypeStr=uint16
  Data Type Conversion5 : DataTypeConversion  OutDataTypeStr=uint16
  FCAN_Send_ID_0xAA : mbd_s32k1xx_ec_toolbox/Communication Blocks/CAN Blocks/FCAN_Send  Priority=2  can_instance=1  can_mode=Non-blocking  can_timeout_ms=0  can_mb_idx=31  can_mb_init=On each call  show_id_input=off  can_extended_id=off  can_is_remote=off  can_id=AA  show_adv_opts=on  can_fd_enable=off  can_enable_brs=on  can_fd_padding=0
  Generate_Data : Subsystem
  Subtract1 : Sum  Inputs=+-
  Subtract2 : Sum  Inputs=+-
  Subtract6 : Sum  Inputs=+-
  SwitchPackRangeOffset{1..5,12} (6 alike) : Constant  Value=SwitchPackRangeOffset  OutDataTypeStr=uint16
  filter : Filter/filter  pwrwndwp_coefcnt=pwrwndwp_coefcnt
  filter1 : Filter/filter  pwrwndwp_coefcnt=pwrwndwp_coefcnt
  filter2 : Filter/filter  pwrwndwp_coefcnt=pwrwndwp_coefcnt
  wires:
  Generate_Data/2(Length) -> FCAN_Send_ID_0xAA/2
  Generate_Data/1(Data) -> FCAN_Send_ID_0xAA/1
  AB_ZC_RearLeftWindowCommand_In1/1 -> filter/1
  AB_ZC_RearRightWindowCommand_In1/1 -> filter1/1
  AB_ZC_PsngrWindowCommand_In1/1 -> filter2/1
  Data Type Conversion5/1 -> Add6/1, Subtract6/1
  Subtract1/1 -> Data Store Write12/1
  Add2/1 -> Data Store Write2/1
  Data Type Conversion2/1 -> Add2/1, Subtract2/1
  SwitchPackRangeOffset2/1 -> Add6/2
  Subtract2/1 -> Data Store Write7/1
  Subtract6/1 -> Data Store Write6/1
  SwitchPackRangeOffset5/1 -> Add1/2
  SwitchPackRangeOffset1/1 -> Subtract6/2
  SwitchPackRangeOffset12/1 -> Add2/2
  Data Type Conversion3/1 -> Add1/1, Subtract1/1
  SwitchPackRangeOffset4/1 -> Subtract2/2
  SwitchPackRangeOffset3/1 -> Subtract1/2
  Add1/1 -> Data Store Write8/1
  Add6/1 -> Data Store Write3/1
  filter/1 -> Data Type Conversion3/1
  filter1/1 -> Data Type Conversion2/1
  filter2/1 -> Data Type Conversion5/1

== system amplifierboard/CAN_Receive_And_Unpack/Subsystem/Chart/CalibrateSwitchPack.SendPos31Response ==
  f : TriggerPort  TriggerType=function-call  VariantControl=(inherit)
      settings: CopyFcn=Stateflow.SLINSF.SimulinkMan.removeBlockPreDeleteFcn  PreDeleteFcn=Stateflow.SLINSF.SimulinkMan.unsafePredeleteFcn
  FCAN_Send_ID_0xAA : mbd_s32k1xx_ec_toolbox/Communication Blocks/CAN Blocks/FCAN_Send  Priority=2  can_instance=1  can_mode=Non-blocking  can_timeout_ms=0  can_mb_idx=31  can_mb_init=On each call  show_id_input=off  can_extended_id=off  can_is_remote=off  can_id=AA  show_adv_opts=on  can_fd_enable=off  can_enable_brs=on  can_fd_padding=0
  Generate_Data : Subsystem
  wires:
  Generate_Data/2(Length) -> FCAN_Send_ID_0xAA/2
  Generate_Data/1(Data) -> FCAN_Send_ID_0xAA/1

== system amplifierboard/CAN_Receive_And_Unpack/Subsystem/Chart/CalibrateSwitchPack.SendPos31Response2 ==
  f : TriggerPort  TriggerType=function-call  VariantControl=(inherit)
      settings: CopyFcn=Stateflow.SLINSF.SimulinkMan.removeBlockPreDeleteFcn  PreDeleteFcn=Stateflow.SLINSF.SimulinkMan.unsafePredeleteFcn
  FCAN_Send_ID_0xAA : mbd_s32k1xx_ec_toolbox/Communication Blocks/CAN Blocks/FCAN_Send  Priority=2  can_instance=1  can_mode=Non-blocking  can_timeout_ms=0  can_mb_idx=30  can_mb_init=On each call  show_id_input=off  can_extended_id=off  can_is_remote=off  can_id=AA  show_adv_opts=on  can_fd_enable=off  can_enable_brs=on  can_fd_padding=0
  Generate_Data : Subsystem
  wires:
  Generate_Data/2(Length) -> FCAN_Send_ID_0xAA/2
  Generate_Data/1(Data) -> FCAN_Send_ID_0xAA/1

== system amplifierboard/CAN_Receive_And_Unpack/Subsystem/Chart/CalibrateSwitchPack.SendPos31StopPosResp ==
  f : TriggerPort  TriggerType=function-call  VariantControl=(inherit)
      settings: CopyFcn=Stateflow.SLINSF.SimulinkMan.removeBlockPreDeleteFcn  PreDeleteFcn=Stateflow.SLINSF.SimulinkMan.unsafePredeleteFcn
  FCAN_Send_ID_0xAA : mbd_s32k1xx_ec_toolbox/Communication Blocks/CAN Blocks/FCAN_Send  Priority=2  can_instance=1  can_mode=Non-blocking  can_timeout_ms=0  can_mb_idx=29  can_mb_init=On each call  show_id_input=off  can_extended_id=off  can_is_remote=off  can_id=AA  show_adv_opts=on  can_fd_enable=off  can_enable_brs=on  can_fd_padding=0
  Generate_Data : Subsystem
  wires:
  Generate_Data/2(Length) -> FCAN_Send_ID_0xAA/2
  Generate_Data/1(Data) -> FCAN_Send_ID_0xAA/1

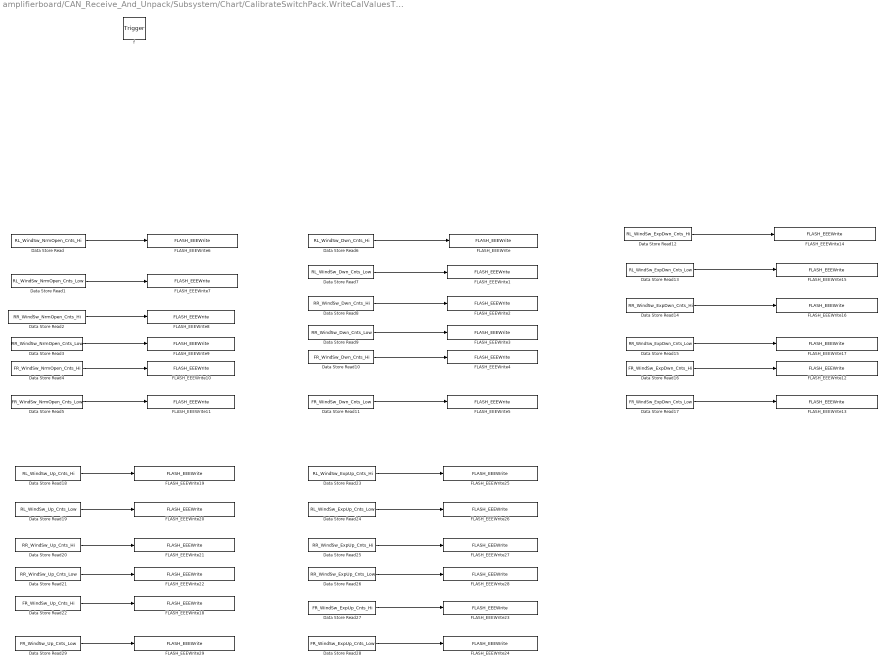
== system amplifierboard/CAN_Receive_And_Unpack/Subsystem/Chart/CalibrateSwitchPack.WriteCalValuesToEEPROM ==
  f : TriggerPort  TriggerType=function-call  VariantControl=(inherit)
      settings: CopyFcn=Stateflow.SLINSF.SimulinkMan.removeBlockPreDeleteFcn  PreDeleteFcn=Stateflow.SLINSF.SimulinkMan.unsafePredeleteFcn
  Data Store Read : DataStoreRead  DataStoreName=RL_WindSw_NrmOpen_Cnts_Hi
  Data Store Read1 : DataStoreRead  DataStoreName=RL_WindSw_NrmOpen_Cnts_Low
  Data Store Read10 : DataStoreRead  DataStoreName=FR_WindSw_Dwn_Cnts_Hi
  Data Store Read11 : DataStoreRead  DataStoreName=FR_WindSw_Dwn_Cnts_Low
  Data Store Read12 : DataStoreRead  DataStoreName=RL_WindSw_ExpDwn_Cnts_Hi
  Data Store Read13 : DataStoreRead  DataStoreName=RL_WindSw_ExpDwn_Cnts_Low
  Data Store Read14 : DataStoreRead  DataStoreName=RR_WindSw_ExpDwn_Cnts_Hi
  Data Store Read15 : DataStoreRead  DataStoreName=RR_WindSw_ExpDwn_Cnts_Low
  Data Store Read16 : DataStoreRead  DataStoreName=FR_WindSw_ExpDwn_Cnts_Hi
  Data Store Read17 : DataStoreRead  DataStoreName=FR_WindSw_ExpDwn_Cnts_Low
  Data Store Read18 : DataStoreRead  DataStoreName=RL_WindSw_Up_Cnts_Hi
  Data Store Read19 : DataStoreRead  DataStoreName=RL_WindSw_Up_Cnts_Low
  Data Store Read2 : DataStoreRead  DataStoreName=RR_WindSw_NrmOpen_Cnts_Hi
  Data Store Read20 : DataStoreRead  DataStoreName=RR_WindSw_Up_Cnts_Hi
  Data Store Read21 : DataStoreRead  DataStoreName=RR_WindSw_Up_Cnts_Low
  Data Store Read22 : DataStoreRead  DataStoreName=FR_WindSw_Up_Cnts_Hi
  Data Store Read23 : DataStoreRead  DataStoreName=RL_WindSw_ExpUp_Cnts_Hi
  Data Store Read24 : DataStoreRead  DataStoreName=RL_WindSw_ExpUp_Cnts_Low
  Data Store Read25 : DataStoreRead  DataStoreName=RR_WindSw_ExpUp_Cnts_Hi
  Data Store Read26 : DataStoreRead  DataStoreName=RR_WindSw_ExpUp_Cnts_Low
  Data Store Read27 : DataStoreRead  DataStoreName=FR_WindSw_ExpUp_Cnts_Hi
  Data Store Read28 : DataStoreRead  DataStoreName=FR_WindSw_ExpUp_Cnts_Low
  Data Store Read29 : DataStoreRead  DataStoreName=FR_WindSw_Up_Cnts_Low
  Data Store Read3 : DataStoreRead  DataStoreName=RR_WindSw_NrmOpen_Cnts_Low
  Data Store Read4 : DataStoreRead  DataStoreName=FR_WindSw_NrmOpen_Cnts_Hi
  Data Store Read5 : DataStoreRead  DataStoreName=FR_WindSw_NrmOpen_Cnts_Low
  Data Store Read6 : DataStoreRead  DataStoreName=RL_WindSw_Dwn_Cnts_Hi
  Data Store Read7 : DataStoreRead  DataStoreName=RL_WindSw_Dwn_Cnts_Low
  Data Store Read8 : DataStoreRead  DataStoreName=RR_WindSw_Dwn_Cnts_Hi
  Data Store Read9 : DataStoreRead  DataStoreName=RR_WindSw_Dwn_Cnts_Low
  FLASH_EEEWrite : mbd_s32k1xx_ec_toolbox/Core and System Blocks/FLASH Blocks/FLASH_EEEWrite  base=0x14000000  offset=0x0F0C  ptr=uint16_t
  FLASH_EEEWrite1 : mbd_s32k1xx_ec_toolbox/Core and System Blocks/FLASH Blocks/FLASH_EEEWrite  base=0x14000000  offset=0x0F0E  ptr=uint16_t
  FLASH_EEEWrite10 : mbd_s32k1xx_ec_toolbox/Core and System Blocks/FLASH Blocks/FLASH_EEEWrite  base=0x14000000  offset=0x0F08  ptr=uint16_t
  FLASH_EEEWrite11 : mbd_s32k1xx_ec_toolbox/Core and System Blocks/FLASH Blocks/FLASH_EEEWrite  base=0x14000000  offset=0x0F0A  ptr=uint16_t
  FLASH_EEEWrite12 : mbd_s32k1xx_ec_toolbox/Core and System Blocks/FLASH Blocks/FLASH_EEEWrite  base=0x14000000  offset=0x0F20  ptr=uint16_t
  FLASH_EEEWrite13 : mbd_s32k1xx_ec_toolbox/Core and System Blocks/FLASH Blocks/FLASH_EEEWrite  base=0x14000000  offset=0x0F22  ptr=uint16_t
  FLASH_EEEWrite14 : mbd_s32k1xx_ec_toolbox/Core and System Blocks/FLASH Blocks/FLASH_EEEWrite  base=0x14000000  offset=0x0F18  ptr=uint16_t
  FLASH_EEEWrite15 : mbd_s32k1xx_ec_toolbox/Core and System Blocks/FLASH Blocks/FLASH_EEEWrite  base=0x14000000  offset=0x0F1A  ptr=uint16_t
  FLASH_EEEWrite16 : mbd_s32k1xx_ec_toolbox/Core and System Blocks/FLASH Blocks/FLASH_EEEWrite  base=0x14000000  offset=0x0F1C  ptr=uint16_t
  FLASH_EEEWrite17 : mbd_s32k1xx_ec_toolbox/Core and System Blocks/FLASH Blocks/FLASH_EEEWrite  base=0x14000000  offset=0x0F1E  ptr=uint16_t
  FLASH_EEEWrite18 : mbd_s32k1xx_ec_toolbox/Core and System Blocks/FLASH Blocks/FLASH_EEEWrite  base=0x14000000  offset=0x0F2C  ptr=uint16_t
  FLASH_EEEWrite19 : mbd_s32k1xx_ec_toolbox/Core and System Blocks/FLASH Blocks/FLASH_EEEWrite  base=0x14000000  offset=0x0F24  ptr=uint16_t
  FLASH_EEEWrite2 : mbd_s32k1xx_ec_toolbox/Core and System Blocks/FLASH Blocks/FLASH_EEEWrite  base=0x14000000  offset=0x0F10  ptr=uint16_t
  FLASH_EEEWrite20 : mbd_s32k1xx_ec_toolbox/Core and System Blocks/FLASH Blocks/FLASH_EEEWrite  base=0x14000000  offset=0x0F26  ptr=uint16_t
  FLASH_EEEWrite21 : mbd_s32k1xx_ec_toolbox/Core and System Blocks/FLASH Blocks/FLASH_EEEWrite  base=0x14000000  offset=0x0F28  ptr=uint16_t
  FLASH_EEEWrite22 : mbd_s32k1xx_ec_toolbox/Core and System Blocks/FLASH Blocks/FLASH_EEEWrite  base=0x14000000  offset=0x0F2A  ptr=uint16_t
  FLASH_EEEWrite23 : mbd_s32k1xx_ec_toolbox/Core and System Blocks/FLASH Blocks/FLASH_EEEWrite  base=0x14000000  offset=0x0F38  ptr=uint16_t
  FLASH_EEEWrite24 : mbd_s32k1xx_ec_toolbox/Core and System Blocks/FLASH Blocks/FLASH_EEEWrite  base=0x14000000  offset=0x0F3A  ptr=uint16_t
  FLASH_EEEWrite25 : mbd_s32k1xx_ec_toolbox/Core and System Blocks/FLASH Blocks/FLASH_EEEWrite  base=0x14000000  offset=0x0F30  ptr=uint16_t
  FLASH_EEEWrite26 : mbd_s32k1xx_ec_toolbox/Core and System Blocks/FLASH Blocks/FLASH_EEEWrite  base=0x14000000  offset=0x0F32  ptr=uint16_t
  FLASH_EEEWrite27 : mbd_s32k1xx_ec_toolbox/Core and System Blocks/FLASH Blocks/FLASH_EEEWrite  base=0x14000000  offset=0x0F34  ptr=uint16_t
  FLASH_EEEWrite28 : mbd_s32k1xx_ec_toolbox/Core and System Blocks/FLASH Blocks/FLASH_EEEWrite  base=0x14000000  offset=0x0F36  ptr=uint16_t
  FLASH_EEEWrite29 : mbd_s32k1xx_ec_toolbox/Core and System Blocks/FLASH Blocks/FLASH_EEEWrite  base=0x14000000  offset=0x0F2E  ptr=uint16_t
  FLASH_EEEWrite3 : mbd_s32k1xx_ec_toolbox/Core and System Blocks/FLASH Blocks/FLASH_EEEWrite  base=0x14000000  offset=0x0F12  ptr=uint16_t
  FLASH_EEEWrite4 : mbd_s32k1xx_ec_toolbox/Core and System Blocks/FLASH Blocks/FLASH_EEEWrite  base=0x14000000  offset=0x0F14  ptr=uint16_t
  FLASH_EEEWrite5 : mbd_s32k1xx_ec_toolbox/Core and System Blocks/FLASH Blocks/FLASH_EEEWrite  base=0x14000000  offset=0x0F16  ptr=uint16_t
  FLASH_EEEWrite6 : mbd_s32k1xx_ec_toolbox/Core and System Blocks/FLASH Blocks/FLASH_EEEWrite  base=0x14000000  offset=0x0F00  ptr=uint16_t
  FLASH_EEEWrite7 : mbd_s32k1xx_ec_toolbox/Core and System Blocks/FLASH Blocks/FLASH_EEEWrite  base=0x14000000  offset=0x0F02  ptr=uint16_t
  FLASH_EEEWrite8 : mbd_s32k1xx_ec_toolbox/Core and System Blocks/FLASH Blocks/FLASH_EEEWrite  base=0x14000000  offset=0x0F04  ptr=uint16_t
  FLASH_EEEWrite9 : mbd_s32k1xx_ec_toolbox/Core and System Blocks/FLASH Blocks/FLASH_EEEWrite  base=0x14000000  offset=0x0F06  ptr=uint16_t
  wires:
  Data Store Read4/1 -> FLASH_EEEWrite10/1
  Data Store Read1/1 -> FLASH_EEEWrite7/1
  Data Store Read2/1 -> FLASH_EEEWrite8/1
  Data Store Read/1 -> FLASH_EEEWrite6/1
  Data Store Read3/1 -> FLASH_EEEWrite9/1
  Data Store Read5/1 -> FLASH_EEEWrite11/1
  Data Store Read6/1 -> FLASH_EEEWrite/1
  Data Store Read11/1 -> FLASH_EEEWrite5/1
  Data Store Read10/1 -> FLASH_EEEWrite4/1
  Data Store Read9/1 -> FLASH_EEEWrite3/1
  Data Store Read7/1 -> FLASH_EEEWrite1/1
  Data Store Read8/1 -> FLASH_EEEWrite2/1
  Data Store Read16/1 -> FLASH_EEEWrite12/1
  Data Store Read12/1 -> FLASH_EEEWrite14/1
  Data Store Read15/1 -> FLASH_EEEWrite17/1
  Data Store Read17/1 -> FLASH_EEEWrite13/1
  Data Store Read13/1 -> FLASH_EEEWrite15/1
  Data Store Read14/1 -> FLASH_EEEWrite16/1
  Data Store Read20/1 -> FLASH_EEEWrite21/1
  Data Store Read21/1 -> FLASH_EEEWrite22/1
  Data Store Read19/1 -> FLASH_EEEWrite20/1
  Data Store Read18/1 -> FLASH_EEEWrite19/1
  Data Store Read22/1 -> FLASH_EEEWrite18/1
  Data Store Read25/1 -> FLASH_EEEWrite27/1
  Data Store Read27/1 -> FLASH_EEEWrite23/1
  Data Store Read24/1 -> FLASH_EEEWrite26/1
  Data Store Read26/1 -> FLASH_EEEWrite28/1
  Data Store Read23/1 -> FLASH_EEEWrite25/1
  Data Store Read28/1 -> FLASH_EEEWrite24/1
  Data Store Read29/1 -> FLASH_EEEWrite29/1

== system amplifierboard/CAN_Receive_And_Unpack/Subsystem/Chart/ECU_Reset ==
  f : TriggerPort  TriggerType=function-call  VariantControl=(inherit)
      settings: CopyFcn=Stateflow.SLINSF.SimulinkMan.removeBlockPreDeleteFcn  PreDeleteFcn=Stateflow.SLINSF.SimulinkMan.unsafePredeleteFcn
  MATLAB Function : MATLAB Function  TreatAsAtomicUnit=on

== system amplifierboard/CAN_Receive_And_Unpack/Subsystem/Chart/InitializeLIN_Cntrler.SendSPI ==
  SPI_Command1 : Inport  OutDataTypeStr=uint8  PortDimensions=[1 10]
  f : TriggerPort  TriggerType=function-call  VariantControl=(inherit)
      settings: CopyFcn=Stateflow.SLINSF.SimulinkMan.removeBlockPreDeleteFcn  PreDeleteFcn=Stateflow.SLINSF.SimulinkMan.unsafePredeleteFcn
  LPSPI_Master_Transfer1 : mbd_s32k1xx_ec_toolbox/Communication Blocks/SPI Blocks/LPSPI_Master_Transfer  instance=0  pcs=0  pcs_polarity=ActiveLow  xfermode=Blocking  timeout=50  spi_upd=on
  LIN_Status10Byte : Outport  OutDataTypeStr=uint8  PortDimensions=[1 10]
  wires:
  SPI_Command1/1 -> LPSPI_Master_Transfer1/1
  LPSPI_Master_Transfer1/1 -> LIN_Status10Byte/1

== system amplifierboard/CAN_Receive_And_Unpack/Subsystem/Chart/InitializeLIN_Cntrler.SendSPI_3Byte ==
  SPI_Command1 : Inport  OutDataTypeStr=uint8  PortDimensions=[1 3]
  f : TriggerPort  TriggerType=function-call  VariantControl=(inherit)
      settings: CopyFcn=Stateflow.SLINSF.SimulinkMan.removeBlockPreDeleteFcn  PreDeleteFcn=Stateflow.SLINSF.SimulinkMan.unsafePredeleteFcn
  LPSPI_Master_Transfer1 : mbd_s32k1xx_ec_toolbox/Communication Blocks/SPI Blocks/LPSPI_Master_Transfer  instance=0  pcs=0  pcs_polarity=ActiveLow  xfermode=Blocking  timeout=50  spi_upd=on
  LIN_Status : Outport  OutDataTypeStr=uint8  PortDimensions=[1 3]
  wires:
  SPI_Command1/1 -> LPSPI_Master_Transfer1/1
  LPSPI_Master_Transfer1/1 -> LIN_Status/1

== system amplifierboard/CAN_Receive_And_Unpack/Subsystem/Chart/InitializeLIN_Cntrler.SendSPI_5Byte ==
  SPI_Command1 : Inport  OutDataTypeStr=uint8  PortDimensions=[1 5]
  f : TriggerPort  TriggerType=function-call  VariantControl=(inherit)
      settings: CopyFcn=Stateflow.SLINSF.SimulinkMan.removeBlockPreDeleteFcn  PreDeleteFcn=Stateflow.SLINSF.SimulinkMan.unsafePredeleteFcn
  LPSPI_Master_Transfer1 : mbd_s32k1xx_ec_toolbox/Communication Blocks/SPI Blocks/LPSPI_Master_Transfer  instance=0  pcs=0  pcs_polarity=ActiveLow  xfermode=Blocking  timeout=50  spi_upd=on
  LIN_Status5Byte : Outport  OutDataTypeStr=uint8  PortDimensions=[1 5]
  wires:
  SPI_Command1/1 -> LPSPI_Master_Transfer1/1
  LPSPI_Master_Transfer1/1 -> LIN_Status5Byte/1

== system amplifierboard/CAN_Receive_And_Unpack/Subsystem/Chart/InitializeLIN_Cntrler1.SendSPI_3Byte ==
  SPI_Command1 : Inport  OutDataTypeStr=uint8  PortDimensions=[1 3]
  f : TriggerPort  TriggerType=function-call  VariantControl=(inherit)
      settings: CopyFcn=Stateflow.SLINSF.SimulinkMan.removeBlockPreDeleteFcn  PreDeleteFcn=Stateflow.SLINSF.SimulinkMan.unsafePredeleteFcn
  LPSPI_Master_Transfer1 : mbd_s32k1xx_ec_toolbox/Communication Blocks/SPI Blocks/LPSPI_Master_Transfer  instance=0  pcs=0  pcs_polarity=ActiveLow  xfermode=Blocking  timeout=50  spi_upd=on
  LIN_Status : Outport  OutDataTypeStr=uint8  PortDimensions=[1 3]
  wires:
  SPI_Command1/1 -> LPSPI_Master_Transfer1/1
  LPSPI_Master_Transfer1/1 -> LIN_Status/1

== system amplifierboard/CAN_Receive_And_Unpack/Subsystem/Chart/SendNeg2EResponse ==
  f : TriggerPort  TriggerType=function-call  VariantControl=(inherit)
      settings: CopyFcn=Stateflow.SLINSF.SimulinkMan.removeBlockPreDeleteFcn  PreDeleteFcn=Stateflow.SLINSF.SimulinkMan.unsafePredeleteFcn
  FCAN_Send_ID_0xAA : mbd_s32k1xx_ec_toolbox/Communication Blocks/CAN Blocks/FCAN_Send  Priority=2  can_instance=1  can_mode=Non-blocking  can_timeout_ms=0  can_mb_idx=31  can_mb_init=On each call  show_id_input=off  can_extended_id=off  can_is_remote=off  can_id=AA  show_adv_opts=on  can_fd_enable=off  can_enable_brs=on  can_fd_padding=0
  Generate_Data : Subsystem
  wires:
  Generate_Data/2(Length) -> FCAN_Send_ID_0xAA/2
  Generate_Data/1(Data) -> FCAN_Send_ID_0xAA/1

== system amplifierboard/CAN_Receive_And_Unpack/Subsystem/Chart/SendPos11Resp ==
  f : TriggerPort  TriggerType=function-call  VariantControl=(inherit)
      settings: CopyFcn=Stateflow.SLINSF.SimulinkMan.removeBlockPreDeleteFcn  PreDeleteFcn=Stateflow.SLINSF.SimulinkMan.unsafePredeleteFcn
  Amplifier_ID_Byte0 : Constant  Value=0x50  OutDataTypeStr=uint8
  Amplifier_ID_Byte1 : Constant  Value=0x72  OutDataTypeStr=uint8
  Amplifier_ID_Byte2 : Constant  Value=0x6F  OutDataTypeStr=uint8  LockScale=on
  Amplifier_ID_Byte3 : Constant  Value=0x67  OutDataTypeStr=uint8  LockScale=on
  Amplifier_ID_Byte4 : Constant  Value=0x69  OutDataTypeStr=uint8
  Amplifier_ID_Byte5 : Constant  Value=0x67  OutDataTypeStr=uint8
  Amplifier_ID_Byte6 : Constant  Value=0x53  OutDataTypeStr=uint8  LockScale=on
  Amplifier_ID_Byte7 : Constant  Value=0x6E  OutDataTypeStr=uint8  LockScale=on
  Amplifier_ID_Byte_10 : mbd_s32k1xx_ec_toolbox/Utility Blocks/DataMemWrite  base=0x1FFFFFF8  offset=0x0002  ptr=uint8_t
  Amplifier_ID_Byte_11 : mbd_s32k1xx_ec_toolbox/Utility Blocks/DataMemWrite  base=0x1FFFFFF8  offset=0x0003  ptr=uint8_t
  Amplifier_ID_Byte_12 : mbd_s32k1xx_ec_toolbox/Utility Blocks/DataMemWrite  base=0x1FFFFFF8  offset=0x0004  ptr=uint8_t
  Amplifier_ID_Byte_13 : mbd_s32k1xx_ec_toolbox/Utility Blocks/DataMemWrite  base=0x1FFFFFF8  offset=0x0005  ptr=uint8_t
  Amplifier_ID_Byte_14 : mbd_s32k1xx_ec_toolbox/Utility Blocks/DataMemWrite  base=0x1FFFFFF8  offset=0x0006  ptr=uint8_t
  Amplifier_ID_Byte_15 : mbd_s32k1xx_ec_toolbox/Utility Blocks/DataMemWrite  base=0x1FFFFFF8  offset=0x0007  ptr=uint8_t
  Amplifier_ID_Byte_8 : mbd_s32k1xx_ec_toolbox/Utility Blocks/DataMemWrite  base=0x1FFFFFF8  offset=0x0000  ptr=uint8_t
  Amplifier_ID_Byte_9 : mbd_s32k1xx_ec_toolbox/Utility Blocks/DataMemWrite  base=0x1FFFFFF8  offset=0x0001  ptr=uint8_t
  FCAN_Send_ID_0xAA : mbd_s32k1xx_ec_toolbox/Communication Blocks/CAN Blocks/FCAN_Send  Priority=2  can_instance=1  can_mode=Non-blocking  can_timeout_ms=0  can_mb_idx=31  can_mb_init=On each call  show_id_input=off  can_extended_id=off  can_is_remote=off  can_id=AA  show_adv_opts=on  can_fd_enable=off  can_enable_brs=on  can_fd_padding=0
  Generate_Data : Subsystem
  wires:
  Generate_Data/1(Data) -> FCAN_Send_ID_0xAA/1
  Generate_Data/2(Length) -> FCAN_Send_ID_0xAA/2
  Amplifier_ID_Byte5/1 -> Amplifier_ID_Byte_14/1
  Amplifier_ID_Byte0/1 -> Amplifier_ID_Byte_8/1
  Amplifier_ID_Byte6/1 -> Amplifier_ID_Byte_12/1
  Amplifier_ID_Byte7/1 -> Amplifier_ID_Byte_15/1
  Amplifier_ID_Byte3/1 -> Amplifier_ID_Byte_11/1
  Amplifier_ID_Byte4/1 -> Amplifier_ID_Byte_13/1
  Amplifier_ID_Byte2/1 -> Amplifier_ID_Byte_10/1
  Amplifier_ID_Byte1/1 -> Amplifier_ID_Byte_9/1

== system amplifierboard/CAN_Receive_And_Unpack/Subsystem/Chart/SendPos22Resp_SW_Ver ==
  f : TriggerPort  TriggerType=function-call  VariantControl=(inherit)
      settings: CopyFcn=Stateflow.SLINSF.SimulinkMan.removeBlockPreDeleteFcn  PreDeleteFcn=Stateflow.SLINSF.SimulinkMan.unsafePredeleteFcn
  FCAN_Send_ID_0xAA : mbd_s32k1xx_ec_toolbox/Communication Blocks/CAN Blocks/FCAN_Send  Priority=2  can_instance=1  can_mode=Non-blocking  can_timeout_ms=0  can_mb_idx=31  can_mb_init=On each call  show_id_input=off  can_extended_id=off  can_is_remote=off  can_id=AA  show_adv_opts=on  can_fd_enable=off  can_enable_brs=on  can_fd_padding=0
  Generate_Data : Subsystem
  wires:
  Generate_Data/1(Data) -> FCAN_Send_ID_0xAA/1
  Generate_Data/2(Length) -> FCAN_Send_ID_0xAA/2

== system amplifierboard/CAN_Receive_And_Unpack/Subsystem/Chart/SendPos22Resp_SW_Ver1 ==
  f : TriggerPort  TriggerType=function-call  VariantControl=(inherit)
      settings: CopyFcn=Stateflow.SLINSF.SimulinkMan.removeBlockPreDeleteFcn  PreDeleteFcn=Stateflow.SLINSF.SimulinkMan.unsafePredeleteFcn
  FCAN_Send_ID_0xAA : mbd_s32k1xx_ec_toolbox/Communication Blocks/CAN Blocks/FCAN_Send  Priority=2  can_instance=1  can_mode=Non-blocking  can_timeout_ms=0  can_mb_idx=31  can_mb_init=On each call  show_id_input=off  can_extended_id=off  can_is_remote=off  can_id=AA  show_adv_opts=on  can_fd_enable=off  can_enable_brs=on  can_fd_padding=0
  Generate_Data : Subsystem
  wires:
  Generate_Data/1(Data) -> FCAN_Send_ID_0xAA/1
  Generate_Data/2(Length) -> FCAN_Send_ID_0xAA/2

== system amplifierboard/CAN_Receive_And_Unpack/Subsystem/Chart/SendPos2EResponse ==
  f : TriggerPort  TriggerType=function-call  VariantControl=(inherit)
      settings: CopyFcn=Stateflow.SLINSF.SimulinkMan.removeBlockPreDeleteFcn  PreDeleteFcn=Stateflow.SLINSF.SimulinkMan.unsafePredeleteFcn
  FCAN_Send_ID_0xAA : mbd_s32k1xx_ec_toolbox/Communication Blocks/CAN Blocks/FCAN_Send  Priority=2  can_instance=1  can_mode=Non-blocking  can_timeout_ms=0  can_mb_idx=31  can_mb_init=On each call  show_id_input=off  can_extended_id=off  can_is_remote=off  can_id=AA  show_adv_opts=on  can_fd_enable=off  can_enable_brs=on  can_fd_padding=0
  Generate_Data : Subsystem
  wires:
  Generate_Data/2(Length) -> FCAN_Send_ID_0xAA/2
  Generate_Data/1(Data) -> FCAN_Send_ID_0xAA/1
